simulink model "engine_with_auto_transmission_test"  (R2026a)
settings: Solver=VariableStepAuto  StopTime=10
libraries: fl_lib x17, nesl_utility x12, sdl_lib x2
settings Model: Creator=doyeop  LastModifiedBy=doyeop

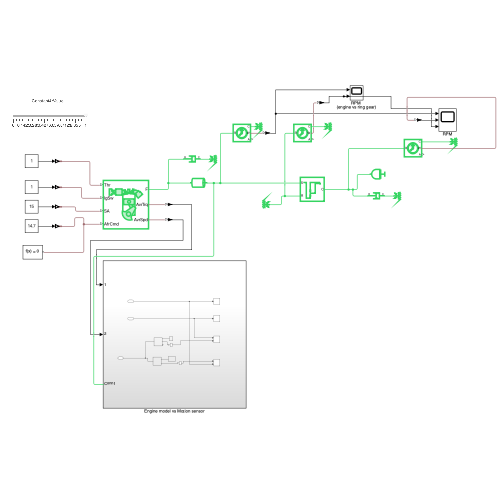
[thumbnail: Simulink's stored preview of the top-level diagram]
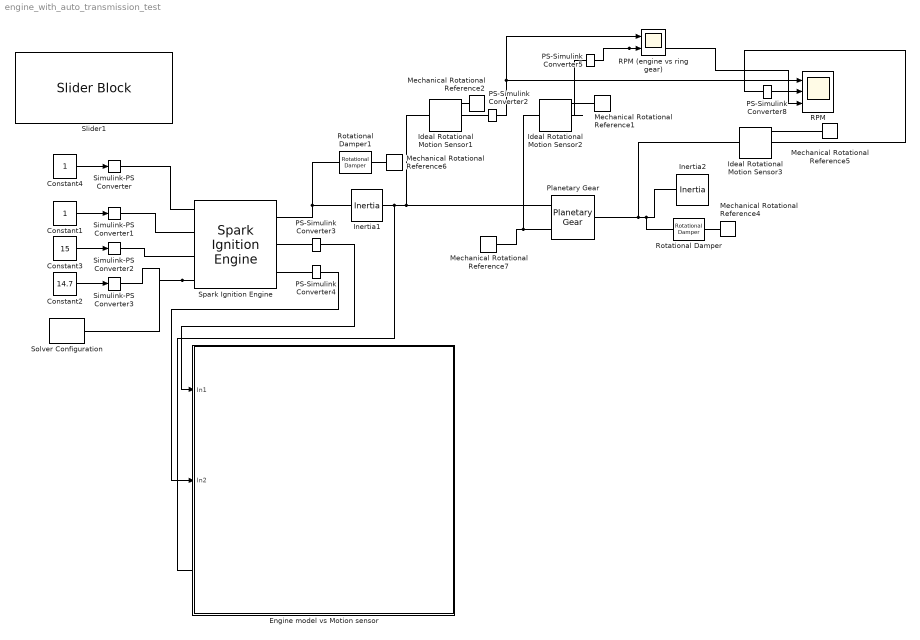
== system engine_with_auto_transmission_test ==
  Constant1 : Constant
  Constant2 : Constant  Value=14.7  SampleTime=-1
  Constant3 : Constant  Value=15  SampleTime=-1
  Constant4 : Constant  SampleTime=-1
  Engine model vs Motion sensor : Subsystem
  Ideal Rotational Motion Sensor1 : fl_lib/Mechanical/Mechanical Sensors/Ideal Rotational Motion Sensor  reference=foundation.enum.MeasurementReference.difference  acceleration_port=false  velocity_port=true  position_port=true  wrap_angle=false  offset=0 rad
  Ideal Rotational Motion Sensor2 : fl_lib/Mechanical/Mechanical Sensors/Ideal Rotational Motion Sensor  reference=foundation.enum.MeasurementReference.difference  acceleration_port=false  velocity_port=true  position_port=true  wrap_angle=false  offset=0 rad
  Ideal Rotational Motion Sensor3 : fl_lib/Mechanical/Mechanical Sensors/Ideal Rotational Motion Sensor  reference=foundation.enum.MeasurementReference.difference  acceleration_port=false  velocity_port=true  position_port=true  wrap_angle=false  offset=0 rad
  Inertia1 : fl_lib/Mechanical/Rotational Elements/Inertia  inertia=0.01 kg*m^2  num_ports=foundation.enum.numPorts2.two  w_specify=on  w_priority=Low  w=800 rpm  w_nominal_specify=off  w_nominal_value=1  w_nominal_unit=rad/s  t_specify=off  t_priority=None  t=0 N*m  t_nominal_specify=off  t_nominal_value=1  t_nominal_unit=N*m
  Inertia2 : fl_lib/Mechanical/Rotational Elements/Inertia  inertia=0.05 kg*m^2  num_ports=foundation.enum.numPorts2.one  w_specify=on  w_priority=None  w=0 rpm  w_nominal_specify=off  w_nominal_value=1  w_nominal_unit=rad/s  t_specify=off  t_priority=None  t=0 N*m  t_nominal_specify=off  t_nominal_value=1  t_nominal_unit=N*m
  Mechanical Rotational Reference{1..2,4..7} (6 alike) : fl_lib/Mechanical/Rotational Elements/Mechanical Rotational Reference
  PS-Simulink Converter{2,4..5,8} (4 alike) : nesl_utility/PS-Simulink Converter  PhysicalDomain=network_engine_domain  SubClassName=ps_output  LeftPortType=input  RightPortType=output  PseudoPeriodic=off  Frequencies=[]  VectorFormat=inherit  Unit=rpm  AffineConversion=off
  PS-Simulink Converter3 : nesl_utility/PS-Simulink Converter  PhysicalDomain=network_engine_domain  SubClassName=ps_output  LeftPortType=input  RightPortType=output  PseudoPeriodic=off  Frequencies=[]  VectorFormat=inherit  Unit=N*m  AffineConversion=off
  Planetary Gear : sdl_lib/Gears/Planetary Gear  rs_ratio=2.4  friction_model=sdl.enum.gear_friction.none  efficiency=[.96, .98]  temperature_TLU=[280, 300, 320] K  efficiency_sp_TLU=[.95, .9, .85]  efficiency_rp_TLU=[.95, .9, .85]  pwr_thr=[.001, .001] W  mu_visc=[0, 0] N*m*s/rad  model_inertia=false  sun_inertia=0.001 kg*m^2  ring_inertia=0.001 kg*m^2  carrier_inertia=0.001 kg*m^2  carrier_radius=0.01 m  planet_inertia=0.001 kg*m^2  planet_mass=0.001 kg  thermal_mass=50 J/K  T_init=300 K
  RPM : Scope  NumInputPorts=3
      settings: ActiveDisplayYMinimum=-545.06879601572211  ActiveDisplayYMaximum=4905.6191641415  DataLoggingVariableName=ScopeData3
  RPM (engine vs ring gear) : Scope  NumInputPorts=2
      settings: ActiveDisplayYMinimum=-1  ActiveDisplayYMaximum=1  DataLoggingVariableName=ScopeData2
  Rotational Damper : fl_lib/Mechanical/Rotational Elements/Rotational Damper  D=0.05 N*m*s/rad  w_specify=off  w_priority=None  w=0 rad/s  w_nominal_specify=off  w_nominal_value=1  w_nominal_unit=rad/s  t_specify=off  t_priority=None  t=0 N*m  t_nominal_specify=off  t_nominal_value=1  t_nominal_unit=N*m
  Rotational Damper1 : fl_lib/Mechanical/Rotational Elements/Rotational Damper  D=0.05 N*m*s/rad  w_specify=off  w_priority=None  w=0 rad/s  w_nominal_specify=off  w_nominal_value=1  w_nominal_unit=rad/s  t_specify=off  t_priority=None  t=0 N*m  t_nominal_specify=off  t_nominal_value=1  t_nominal_unit=N*m
  Simulink-PS Converter : nesl_utility/Simulink-PS Converter  PhysicalDomain=network_engine_domain  SubClassName=ps_input  LeftPortType=input  RightPortType=output  PseudoPeriodic=off  Frequencies=[]  NoiseDistribution=none  NoiseParameters=[]  Unit=1  AffineConversion=off  FilteringAndDerivatives=provide  SimscapeFilterOrder=1  InputFilterTimeConstant=0.001  UdotUserProvided=0
  Simulink-PS Converter1 : nesl_utility/Simulink-PS Converter  PhysicalDomain=network_engine_domain  SubClassName=ps_input  LeftPortType=input  RightPortType=output  PseudoPeriodic=off  Frequencies=[]  NoiseDistribution=none  NoiseParameters=[]  Unit=1  AffineConversion=off  FilteringAndDerivatives=provide  SimscapeFilterOrder=1  InputFilterTimeConstant=0.001  UdotUserProvided=0
  Simulink-PS Converter2 : nesl_utility/Simulink-PS Converter  PhysicalDomain=network_engine_domain  SubClassName=ps_input  LeftPortType=input  RightPortType=output  PseudoPeriodic=off  Frequencies=[]  NoiseDistribution=none  NoiseParameters=[]  Unit=deg  AffineConversion=off  FilteringAndDerivatives=provide  SimscapeFilterOrder=1  InputFilterTimeConstant=0.001  UdotUserProvided=0
  Simulink-PS Converter3 : nesl_utility/Simulink-PS Converter  PhysicalDomain=network_engine_domain  SubClassName=ps_input  LeftPortType=input  RightPortType=output  PseudoPeriodic=off  Frequencies=[]  NoiseDistribution=none  NoiseParameters=[]  Unit=1  AffineConversion=off  FilteringAndDerivatives=provide  SimscapeFilterOrder=1  InputFilterTimeConstant=0.001  UdotUserProvided=0
  Slider1 : SliderBlock  ScaleMax=1
  Solver Configuration : nesl_utility/Solver Configuration  PhysicalDomain=network_engine_domain  SubClassName=solver  LeftPortType=input  RightPortType=generic  Tones=[]  Harmonics=[]  SimulateNoise=off  Profile=off  UseLocalSampling=off  EnableSwitchedLinearOptims=on  FrequencyDomain=off  UseCCode=off  RelTol=0.001  AbsTol=0.001  MinStep=1e-09  ToWorkspace=off  RevertToSquareIcSolve=off  NumHomotopyIterations=100  PhasorMode=off  PhasorModeNumHarmonics=1  ConsistencySolver=NEWTON_XTOL_AFTER_FTOL  CanonicalOrdering=CANONICAL  OptimizeIntermediates=OPTIMIZED  IndexReductionMethod=DerivativeReplacement  DoDC=off  ResidualTolerance=1e-09  ConsistencyTolSource=GLOBAL  ConsistencyAbsTol=0.001  ConsistencyRelTol=0.001  ConsistencyTolFactor=0.001  UseLocalSolver=off  LocalSolverChoice=NE_BACKWARD_EULER_ADVANCER  ResolveIndetEquations=on  FunctionEvalNumThread=1  LocalSolverSampleTime=0.001  DoFixedCost=off  MaxNonlinIter=3  MaxModeIter=2  ComputeImpulses=off  ImpulseIterations=2  LinearAlgebra=auto  LinearAlgebraNumThread=0  EquationFormulation=NE_TIME_EF  DelaysMemoryBudget=1024  AutomaticFiltering=on  FilteringTimeConstant=0.001  PartitionStorageMethod=AS_NEEDED  PartitionMemoryBudget=1024  PartitionMethod=ROBUST  MultibodyUseLocalSolver=off  MultibodyLocalSolverChoice=ODE1  MultibodyLocalSolverSampleTime=0.001
  Spark Ignition Engine : sdl_lib/Engines & Motors/Spark Ignition Engine  numCyls=sdl.enum.engineNumCylinders.Four  twoCylSADiff=270 deg  L4FiringOrder=sdl.enum.engineFiringOrderFourCylinders.L4_1342  bore=67 mm  stroke=42.5 mm  conrod=90 mm  CR=12.2  P_amb=101.325 kPa  T_amb=298.15 K  rho_air=1.225 mg/cm^3  R_air=288.1965 J/(K*kg)  UseAirIntake=true  c_thr=0.1 s  thr_rest=3 deg  D_plate=5 cm  S_leak=1 cm^2  V_im=500 cm^3  Cd_in=0.9  IVO_0=-10 deg  IVC_0=100 deg  EVO_0=30 deg  EVC_0=5 deg  UseInVVT=false  UseExVVT=false  q_LHV=44.3 MJ/kg  InputAFR=true  AFR_const=14.6  InputInjPw=false  Sinj=6.5 mg/ms  SparkInputType=sdl.enum.engineSparkInputType.Angle  SA_const=20 deg  comb_bd=50 deg  dt_Pcyl_slow_decay=60 s  dt_Tcyl_slow_decay=600 s  dt_exh_decay=5 ms  InputBackPressure=false  dP_exh=50 kPa  dw_exh=6000 rpm  UseExhaustThermal=true  S_exh=1 m^2  M_exh=5 kg  C_exh=100 J/(K*kg)  k_gas=10 s  h_convection=100 W/(K*m^2)  k_radiation=0.3  SB=5.7e-8 W/(K^4*m^2)  Pim_0=101.325 kPa  ca0=0 deg  w0=800 rpm  EngSpdSimLimit=16000 rpm  OutputTorqueAvr=true  OutputSpeedAvr=true  OutputCrkpos=false  OutputPim=false  OutputAirMassFlow=false  OutputFuelMassFlow=false  OutputAFR=false  OutputVcyl=false  OutputPcyl=false  OutputTcyl=false  OutputTexh=false
  wires:
  Constant2/1 -> Simulink-PS Converter3/1
  Constant3/1 -> Simulink-PS Converter2/1
  Constant4/1 -> Simulink-PS Converter/1
  Constant1/1 -> Simulink-PS Converter1/1
  PS-Simulink Converter2/1 -> RPM (engine vs ring gear)/1, RPM/1
  PS-Simulink Converter5/1 -> RPM/3, RPM (engine vs ring gear)/2
  PS-Simulink Converter8/1 -> RPM/2
  PS-Simulink Converter3/1 -> Engine model vs Motion sensor/1(In1)
  PS-Simulink Converter4/1 -> Engine model vs Motion sensor/2(In2)
  connections:
  Spark Ignition Engine/LConn4 -- Simulink-PS Converter3/RConn1 -- Solver Configuration/RConn1
  Simulink-PS Converter2/RConn1 -- Spark Ignition Engine/LConn3
  Simulink-PS Converter1/RConn1 -- Spark Ignition Engine/LConn2
  PS-Simulink Converter3/LConn1 -- Spark Ignition Engine/RConn2
  Simulink-PS Converter/RConn1 -- Spark Ignition Engine/LConn1
  Inertia1/RConn1 -- Spark Ignition Engine/RConn1 -- Rotational Damper1/LConn1
  PS-Simulink Converter4/LConn1 -- Spark Ignition Engine/RConn3
  PS-Simulink Converter2/LConn1 -- Ideal Rotational Motion Sensor1/RConn2
  Mechanical Rotational Reference2/LConn1 -- Ideal Rotational Motion Sensor1/RConn1
  Mechanical Rotational Reference4/LConn1 -- Rotational Damper/RConn1
  Ideal Rotational Motion Sensor3/RConn2 -- PS-Simulink Converter8/LConn1
  Mechanical Rotational Reference5/LConn1 -- Ideal Rotational Motion Sensor3/RConn1
  Mechanical Rotational Reference6/LConn1 -- Rotational Damper1/RConn1
  Planetary Gear/RConn2 -- Engine model vs Motion sensor/LConn1 -- Inertia1/LConn1 -- Ideal Rotational Motion Sensor1/LConn1
  Ideal Rotational Motion Sensor2/RConn2 -- PS-Simulink Converter5/LConn1
  Mechanical Rotational Reference1/LConn1 -- Ideal Rotational Motion Sensor2/RConn1
  Planetary Gear/LConn1 -- Inertia2/LConn1 -- Rotational Damper/LConn1 -- Ideal Rotational Motion Sensor3/LConn1
  Ideal Rotational Motion Sensor2/LConn1 -- Planetary Gear/RConn1 -- Mechanical Rotational Reference7/LConn1

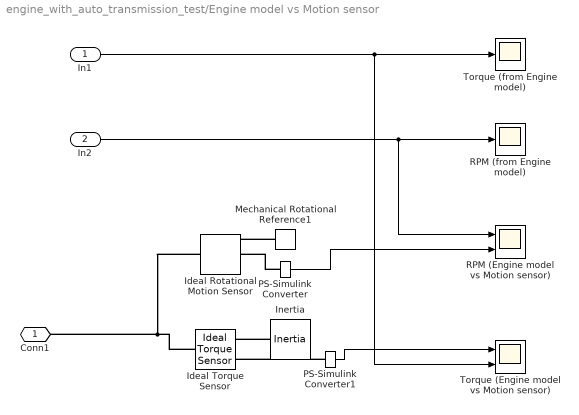
== system engine_with_auto_transmission_test/Engine model vs Motion sensor ==
  In1 : Inport
  In2 : Inport  Port=2
  Ideal Rotational Motion Sensor : fl_lib/Mechanical/Mechanical Sensors/Ideal Rotational Motion Sensor  reference=foundation.enum.MeasurementReference.difference  acceleration_port=false  velocity_port=true  position_port=true  wrap_angle=false  offset=0 rad
  Ideal Torque Sensor : fl_lib/Mechanical/Mechanical Sensors/Ideal Torque Sensor
  Inertia : fl_lib/Mechanical/Rotational Elements/Inertia  inertia=0.1 kg*m^2  num_ports=foundation.enum.numPorts2.one  w_specify=on  w_priority=None  w=0 rpm  w_nominal_specify=off  w_nominal_value=1  w_nominal_unit=rad/s  t_specify=off  t_priority=None  t=0 N*m  t_nominal_specify=off  t_nominal_value=1  t_nominal_unit=N*m
  Mechanical Rotational Reference1 : fl_lib/Mechanical/Rotational Elements/Mechanical Rotational Reference
  PS-Simulink Converter : nesl_utility/PS-Simulink Converter  PhysicalDomain=network_engine_domain  SubClassName=ps_output  LeftPortType=input  RightPortType=output  PseudoPeriodic=off  Frequencies=[]  VectorFormat=inherit  Unit=rpm  AffineConversion=off
  PS-Simulink Converter1 : nesl_utility/PS-Simulink Converter  PhysicalDomain=network_engine_domain  SubClassName=ps_output  LeftPortType=input  RightPortType=output  PseudoPeriodic=off  Frequencies=[]  VectorFormat=inherit  Unit=N*m  AffineConversion=off
  RPM (Engine model vs Motion sensor) : Scope  NumInputPorts=2
      settings: ActiveDisplayYMinimum=-419.44946675369869  ActiveDisplayYMaximum=3775.0452007832891
  RPM (from Engine model) : Scope
      settings: ActiveDisplayYMinimum=-545.70228379071159  ActiveDisplayYMaximum=4911.3205541164052  DataLoggingVariableName=ScopeData6
  Torque (Engine model vs Motion sensor) : Scope  NumInputPorts=2
      settings: ActiveDisplayYMinimum=-41.551396950603035  ActiveDisplayYMaximum=102.79160135138113
  Torque (from Engine model) : Scope
      settings: ActiveDisplayYMinimum=-2.7967171219384035  ActiveDisplayYMaximum=25.170454097445635  DataLoggingVariableName=ScopeData5
  Conn1 : PMIOPort  Side=Left
  wires:
  PS-Simulink Converter/1 -> RPM (Engine model vs Motion sensor)/2
  In2/1 -> RPM (from Engine model)/1, RPM (Engine model vs Motion sensor)/1
  In1/1 -> Torque (Engine model vs Motion sensor)/2, Torque (from Engine model)/1
  PS-Simulink Converter1/1 -> Torque (Engine model vs Motion sensor)/1
  connections:
  PS-Simulink Converter1/LConn1 -- Ideal Torque Sensor/RConn2
  Mechanical Rotational Reference1/LConn1 -- Ideal Rotational Motion Sensor/RConn1
  PS-Simulink Converter/LConn1 -- Ideal Rotational Motion Sensor/RConn2
  Ideal Torque Sensor/LConn1 -- Ideal Rotational Motion Sensor/LConn1 -- Conn1/RConn1
  Inertia/LConn1 -- Ideal Torque Sensor/RConn1
